simulink model "Passive_Cell_Balancing"  (R2024b)
settings: Solver=VariableStepAuto  StartTime=0.0  StopTime=1200  RelTol=1e-3
undefined symbols (not defined in the file): Ion, Lithium
libraries: spsSeriesRLCBranchLib x4, spsBatteryLib x3, spsIGBTDiodeLib x3, spsIdealSwitchLib x2, spsDCVoltageSourceLib x1, spsGroundLib x1, sps_lib x1
settings Model: Creator=harsh

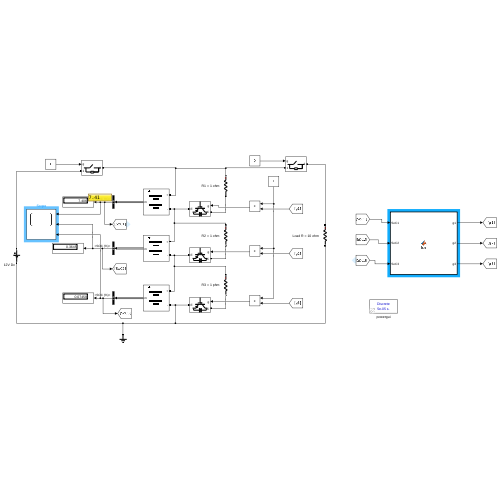
[thumbnail: Simulink's stored preview of the top-level diagram]
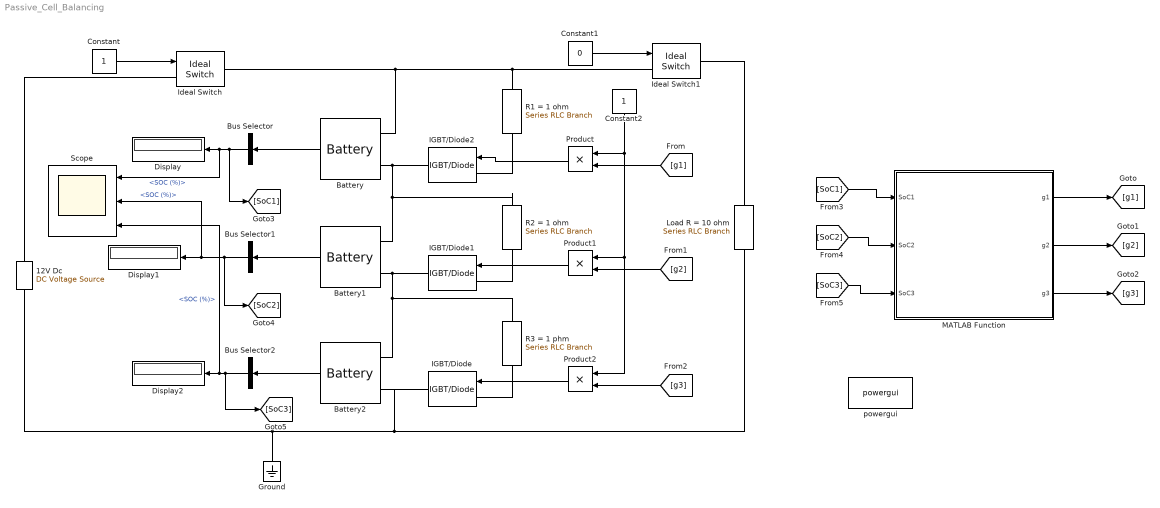
== system Passive_Cell_Balancing ==
  "12V Dc               " : spsDCVoltageSourceLib/DC Voltage Source  Amplitude=12  Measurements=None
  Battery : spsBatteryLib/Battery  BatType=Lithium-Ion  NomV=3.7  NomQ=5.4  SOC=60  Batt_Tr=30  PresetModel=on  MaxQ=5.4  MinV=2.775  FullV=4.3068  Dis_rate=2.3478  R=0.0068519  Normal_OP=4.8835  expZone="[3.9974      0.2653]"
  Battery1 : spsBatteryLib/Battery  BatType=Lithium-Ion  NomV=3.7  NomQ=5.4  SOC=50  Batt_Tr=30  PresetModel=on  MaxQ=5.4  MinV=2.775  FullV=4.3068  Dis_rate=2.3478  R=0.0068519  Normal_OP=4.8835  expZone="[3.9974      0.2653]"
  Battery2 : spsBatteryLib/Battery  BatType=Lithium-Ion  NomV=3.7  NomQ=5.4  SOC=40  Batt_Tr=10  PresetModel=on  MaxQ=5.4  MinV=2.775  FullV=4.3068  Dis_rate=2.3478  R=0.0068519  Normal_OP=4.8835  expZone="[3.9974      0.2653]"
  Bus Selector : BusSelector  OutputSignals=SOC (%)
  Bus Selector1 : BusSelector  OutputSignals=SOC (%)
  Bus Selector2 : BusSelector  OutputSignals=SOC (%)
  Constant : Constant
  Constant1 : Constant  Value=0
  Constant2 : Constant
  Display : Display
  Display1 : Display
  Display2 : Display
  Ground : spsGroundLib/Ground  LConnTagsString=a
  IGBT/Diode : spsIGBTDiodeLib/IGBT//Diode  Ron=1e-3  Rs=1e5  Cs=inf  Measurements=off
  IGBT/Diode1 : spsIGBTDiodeLib/IGBT//Diode  Ron=1e-3  Rs=1e5  Cs=inf  Measurements=off
  IGBT/Diode2 : spsIGBTDiodeLib/IGBT//Diode  Ron=1e-3  Rs=1e5  Cs=inf  Measurements=off
  Ideal Switch : spsIdealSwitchLib/Ideal Switch  Ron=0.001  Lon=0  IC=0  Rs=1e5  Cs=inf  Measurements=off
  Ideal Switch1 : spsIdealSwitchLib/Ideal Switch  Ron=0.001  Lon=0  IC=0  Rs=1e5  Cs=inf  Measurements=off
  Load R = 10 ohm : spsSeriesRLCBranchLib/Series RLC Branch  LConnTagsString=__new0  RConnTagsString=__new0  BranchType=R  Resistance=10  Inductance=1e-3  SetiL0=off  InitialCurrent=0  Capacitance=1e-6  Setx0=off  InitialVoltage=0  Measurements=None
  MATLAB Function : MATLAB Function  TreatAsAtomicUnit=on
  Product : Product
  Product1 : Product
  Product2 : Product
  R1 = 1 ohm : spsSeriesRLCBranchLib/Series RLC Branch  LConnTagsString=__new0  RConnTagsString=__new0  BranchType=R  Resistance=1  Inductance=1e-3  SetiL0=off  InitialCurrent=0  Capacitance=1e-6  Setx0=off  InitialVoltage=0  Measurements=None
  R2 = 1 ohm : spsSeriesRLCBranchLib/Series RLC Branch  LConnTagsString=__new0  RConnTagsString=__new0  BranchType=R  Resistance=1  Inductance=1e-3  SetiL0=off  InitialCurrent=0  Capacitance=1e-6  Setx0=off  InitialVoltage=0  Measurements=None
  R3 = 1 phm : spsSeriesRLCBranchLib/Series RLC Branch  LConnTagsString=__new0  RConnTagsString=__new0  BranchType=R  Resistance=1  Inductance=1e-3  SetiL0=off  InitialCurrent=0  Capacitance=1e-6  Setx0=off  InitialVoltage=0  Measurements=None
  Scope : Scope  NumInputPorts=3
  powergui : sps_lib/powergui  Priority=1  SimulationMode=Discrete  SampleTime=50e-6  frequency=60  Iterations=50  frequencyindice=0  Pbase=100e6  ErrMax=1e-4  UnitsV=kV  UnitsW=MW  buscounter=0  FunctionMessages=off  echomessages=off  EnableUseOfTLC=off  CurrentSourceSwitches=off  DisableSnubberDevices=off  DisableRonSwitches=off  DisableVfSwitches=off  DisplayEquations=off  AutomaticDiscreteSolvers=off  SolverType=Tustin/Backward Euler (TBE)  Interpol=off  ExternalGateDelay=off  methode=off  Ts=100  x0status=blocks  SPID=on  SwTol=0  HookPort=off  NonlinearTolerance=1e-4  nMaxIteration=100  ContinueOnMaxIteration=off  RestoreLinks=warning  ResistiveCurrentMeasurement=off  Frange=[0:2:500]  Ylog=off  Xlog=on  ShowGrid=off  save=off  variable=ZData  structure=0  ZoomFFT=off  StartTime=0.0  cycles=1  DisplayStyle=1  fundamental=60  FreqAxis=off  MaxFrequency=1000  frequencyindicesteady=1  RmsSteady=1  display=off
  wires:
  Constant/1 -> Ideal Switch/1
  Constant1/1 -> Ideal Switch1/1
  Battery/1 -> Bus Selector/1
  Bus Selector/1 -> [SoC1], Scope/1, Display/1  "<SOC (%)>"
  Bus Selector1/1 -> [SoC2], Scope/2, Display1/1  "<SOC (%)>"
  Battery1/1 -> Bus Selector1/1
  Battery2/1 -> Bus Selector2/1
  Bus Selector2/1 -> [SoC3], Scope/3, Display2/1  "<SOC (%)>"
  Constant2/1 -> Product/1, Product1/1, Product2/1
  [g1] -> Product/2
  [g2] -> Product1/2
  [g3] -> Product2/2
  Product/1 -> IGBT/Diode2/1
  Product1/1 -> IGBT/Diode1/1
  Product2/1 -> IGBT/Diode/1
  MATLAB Function/1(g1) -> [g1]
  MATLAB Function/2(g2) -> [g2]
  MATLAB Function/3(g3) -> [g3]
  [SoC1] -> MATLAB Function/1(SoC1)
  [SoC2] -> MATLAB Function/2(SoC2)
  [SoC3] -> MATLAB Function/3(SoC3)
  connections:
  Battery1/LConn2 -- IGBT/Diode1/RConn1 -- R3 = 1 phm/LConn1 -- Battery2/LConn1
  Battery/LConn2 -- IGBT/Diode2/RConn1 -- R2 = 1 ohm/LConn1 -- Battery1/LConn1
  IGBT/Diode/LConn1 -- R3 = 1 phm/RConn1
  IGBT/Diode1/LConn1 -- R2 = 1 ohm/RConn1
  IGBT/Diode2/LConn1 -- R1 = 1 ohm/RConn1
  R1 = 1 ohm/LConn1 -- Ideal Switch1/LConn1 -- Battery/LConn1 -- Ideal Switch/RConn1
  "12V Dc               "/RConn1 -- Ideal Switch/LConn1
  Load R = 10 ohm/RConn1 -- IGBT/Diode/RConn1 -- Battery2/LConn2 -- Ground/LConn1 -- "12V Dc               "/LConn1
  Load R = 10 ohm/LConn1 -- Ideal Switch1/RConn1

== matlab function Passive_Cell_Balancing/MATLAB Function ==
  data: SoC1 input; g1 output; SoC2 input; SoC3 input; g2 output; g3 output
function [g1,g2,g3] = fcn(SoC1,SoC2,SoC3)

SoC1=int32(SoC1);
SoC2=int32(SoC2);
SoC3=int32(SoC3);
 
if SoC1>SoC2||SoC1>SoC3
    g1=1;
else 
    g1=0;
end
if SoC2>SoC1||SoC2>SoC3
    g2=1;
else
    g2=0;
end 
if SoC3>SoC1||SoC3>SoC2
g3=1;
else 
    g3=0;
end
